simulink model "Task3_DSB_Sim"  (R2024b)
settings: Solver=FixedStepDiscrete  StartTime=0.0  StopTime=0.01  FixedStep=1/100000  RelTol=1e-3
libraries: simulink_extras x18, dspsrcs4 x6, commanapbnd3 x4, commchan3 x2
settings Model: Creator=kbali  LastModifiedBy=kbali

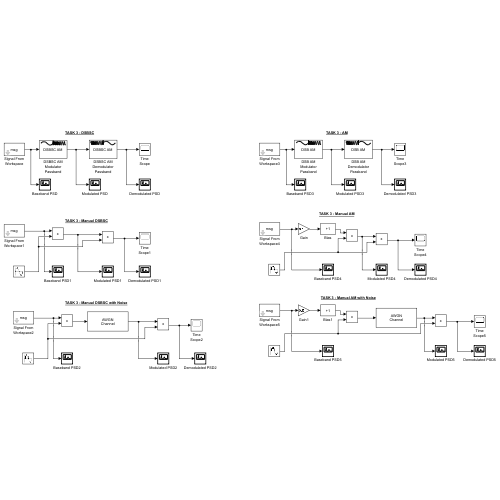
[thumbnail: Simulink's stored preview of the top-level diagram]
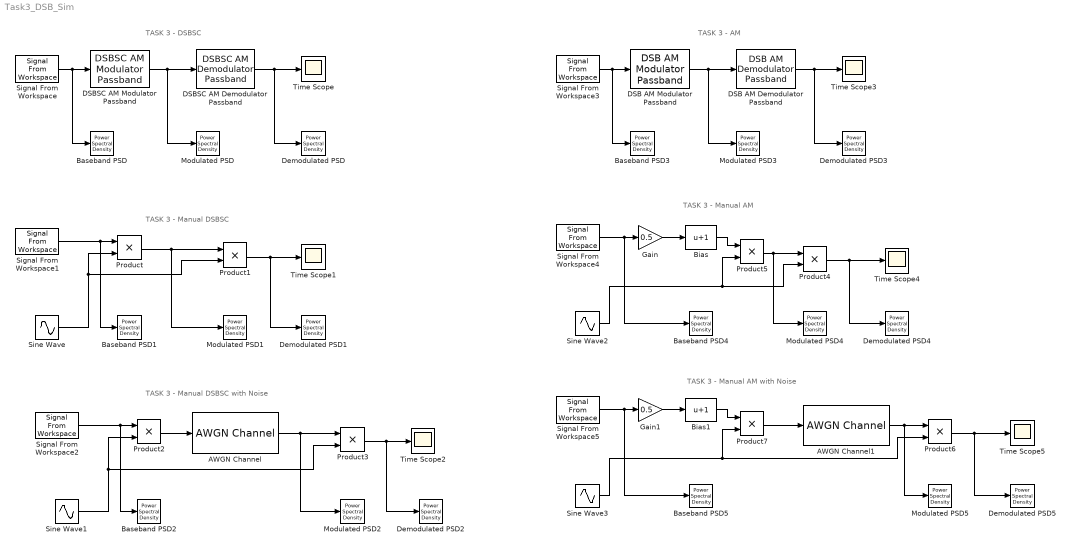
== system Task3_DSB_Sim ==
  note: TASK 3 - DSBSC
  note: TASK 3 - Manual DSBSC
  note: TASK 3 - Manual DSBSC with Noise
  note: TASK 3 - AM
  note: TASK 3 - Manual AM
  note: TASK 3 - Manual AM with Noise
  AWGN Channel : commchan3/AWGN Channel  LegacyMode=off  NoiseMethod="Signal to noise ratio  (SNR)"  noiseMode="Signal to noise ratio  (SNR)"  EbNo=10  EsNo=10  SNR=0  BitsPerSymbol=1  SignalPower=1  SamplesPerSymbol=1  SymbolPeriod=1  VarianceSource=Parameter  Variance=1  RandomStream=Global stream  Seed=67  SimulateUsing=Code generation
  AWGN Channel1 : commchan3/AWGN Channel  LegacyMode=off  NoiseMethod="Signal to noise ratio  (SNR)"  noiseMode="Signal to noise ratio  (SNR)"  EbNo=10  EsNo=10  SNR=0  BitsPerSymbol=1  SignalPower=1  SamplesPerSymbol=1  SymbolPeriod=1  VarianceSource=Parameter  Variance=1  RandomStream=Global stream  Seed=67  SimulateUsing=Code generation
  Baseband PSD{,1..5} (6 alike) : simulink_extras/Additional Sinks/Power Spectral Density  npts=128  fftpts=512  HowOften=64  sampleT=0.00001
  Bias : Bias  Bias=1  SaturateOnIntegerOverflow=off
  Bias1 : Bias  Bias=1  SaturateOnIntegerOverflow=off
  DSB AM Demodulator Passband : commanapbnd3/DSB AM Demodulator Passband  Fc=10000  Ph=0  method=Butterworth  n=4  cf=2000  Rp=0.1  Rs=50  Offset=1
  DSB AM Modulator Passband : commanapbnd3/DSB AM Modulator Passband  Fc=10000  Ph=0  Offset=1
  DSBSC AM Demodulator Passband : commanapbnd3/DSBSC AM Demodulator Passband  Fc=10000  Ph=0  method=Butterworth  n=4  cf=2000  Rp=0.1  Rs=50
  DSBSC AM Modulator Passband : commanapbnd3/DSBSC AM Modulator Passband  Fc=10000  Ph=0
  Demodulated PSD{,1..5} (6 alike) : simulink_extras/Additional Sinks/Power Spectral Density  npts=128  fftpts=512  HowOften=64  sampleT=0.00001
  Gain : Gain  Gain=0.5
  Gain1 : Gain  Gain=0.5
  Modulated PSD{,1..5} (6 alike) : simulink_extras/Additional Sinks/Power Spectral Density  npts=128  fftpts=512  HowOften=64  sampleT=0.00001
  Product{,1..7} (8 alike) : Product
  Signal From Workspace{,1..5} (6 alike) : dspsrcs4/Signal From Workspace  X=msg  Ts=1/100000  nsamps=1  OutputAfterFinalValue=Setting to zero  ignoreOrWarnInputAndFrameLengths=off  OutputFrames=off
  Sine Wave{,1..3} (4 alike) : Sin  Frequency=2*pi*10000  SampleTime=1/100000
  Time Scope{,1..5} (6 alike) : Scope
  wires:
  DSBSC AM Modulator Passband/1 -> Modulated PSD/1, DSBSC AM Demodulator Passband/1
  Signal From Workspace/1 -> Baseband PSD/1, DSBSC AM Modulator Passband/1
  DSBSC AM Demodulator Passband/1 -> Demodulated PSD/1, Time Scope/1
  Sine Wave/1 -> Product1/2, Product/2
  Signal From Workspace1/1 -> Baseband PSD1/1, Product/1
  Product/1 -> Modulated PSD1/1, Product1/1
  Product1/1 -> Demodulated PSD1/1, Time Scope1/1
  Sine Wave1/1 -> Product3/2, Product2/2
  Signal From Workspace2/1 -> Baseband PSD2/1, Product2/1
  Product2/1 -> AWGN Channel/1
  AWGN Channel/1 -> Modulated PSD2/1, Product3/1
  Product3/1 -> Demodulated PSD2/1, Time Scope2/1
  DSB AM Demodulator Passband/1 -> Demodulated PSD3/1, Time Scope3/1
  DSB AM Modulator Passband/1 -> DSB AM Demodulator Passband/1, Modulated PSD3/1
  Signal From Workspace3/1 -> DSB AM Modulator Passband/1, Baseband PSD3/1
  Signal From Workspace4/1 -> Baseband PSD4/1, Gain/1
  Gain/1 -> Bias/1
  Bias/1 -> Product5/1
  Sine Wave2/1 -> Product4/2, Product5/2
  Product5/1 -> Modulated PSD4/1, Product4/1
  Product4/1 -> Demodulated PSD4/1, Time Scope4/1
  Product6/1 -> Demodulated PSD5/1, Time Scope5/1
  Bias1/1 -> Product7/1
  Gain1/1 -> Bias1/1
  Sine Wave3/1 -> Product6/2, Product7/2
  Signal From Workspace5/1 -> Baseband PSD5/1, Gain1/1
  Product7/1 -> AWGN Channel1/1
  AWGN Channel1/1 -> Modulated PSD5/1, Product6/1
